simulink model "ZOH_ie"  (R2018b)
settings: Solver=VariableStepAuto  StartTime=0.0  StopTime=20  MaxStep=0.01  RelTol=1e-3
settings Model: EnablePacing=on  PacingRate=0.710000  Creator=td  LastModifiedBy=td

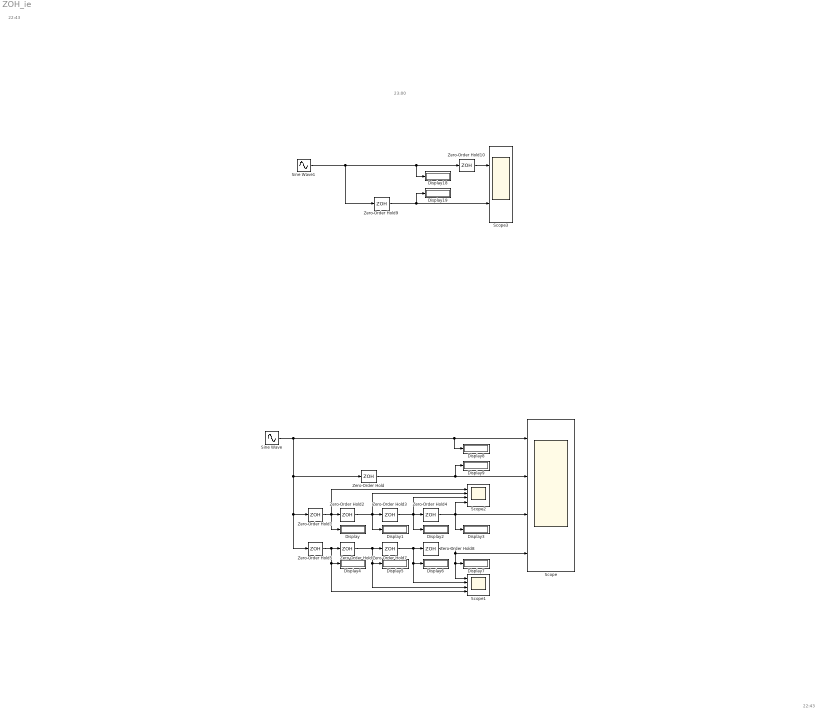
== system ZOH_ie ==
  note: 23:00
  note: 22:43
  note: 22:43
  Display{,1..9,18..19} (12 alike) : Display
  Scope : Scope  NumInputPorts=4
  Scope1 : Scope  NumInputPorts=4
  Scope2 : Scope  NumInputPorts=4
  Scope3 : Scope  NumInputPorts=2
  Sine Wave : Sin  SampleTime=0
  Sine Wave1 : Sin  SampleTime=0
  Zero-Order Hold{,1..4,9..10} (7 alike) : ZeroOrderHold
  Zero-Order Hold5 : ZeroOrderHold  SampleTime=0.9
  Zero-Order Hold6 : ZeroOrderHold  SampleTime=0.8
  Zero-Order Hold7 : ZeroOrderHold  SampleTime=0.7
  Zero-Order Hold8 : ZeroOrderHold  SampleTime=0.6
  wires:
  Sine Wave/1 -> Zero-Order Hold5/1, Zero-Order Hold1/1, Zero-Order Hold/1, Display8/1, Scope/1
  Zero-Order Hold/1 -> Display9/1, Scope/2
  Zero-Order Hold1/1 -> Scope2/1, Zero-Order Hold2/1, Display/1
  Zero-Order Hold2/1 -> Scope2/2, Display1/1, Zero-Order Hold3/1
  Zero-Order Hold3/1 -> Scope2/3, Display2/1, Zero-Order Hold4/1
  Zero-Order Hold4/1 -> Scope2/4, Display3/1, Scope/3
  Zero-Order Hold7/1 -> Scope1/2, Display6/1, Zero-Order Hold8/1
  Zero-Order Hold6/1 -> Scope1/3, Display5/1, Zero-Order Hold7/1
  Zero-Order Hold5/1 -> Scope1/4, Display4/1, Zero-Order Hold6/1
  Zero-Order Hold8/1 -> Scope1/1, Display7/1, Scope/4
  Zero-Order Hold9/1 -> Display19/1, Scope3/2
  Sine Wave1/1 -> Zero-Order Hold9/1, Zero-Order Hold10/1, Display18/1
  Zero-Order Hold10/1 -> Scope3/1
